simulink model "AERO560_HW6Sim_Thapar"  (R2022b)
settings: Solver=VariableStepAuto  StartTime=0.0  StopTime=10.0  RelTol=1e-3
undefined symbols (not defined in the file): p1, seed
settings Model: Creator=gagandeepthapar  LastModifiedBy=gagandeepthapar

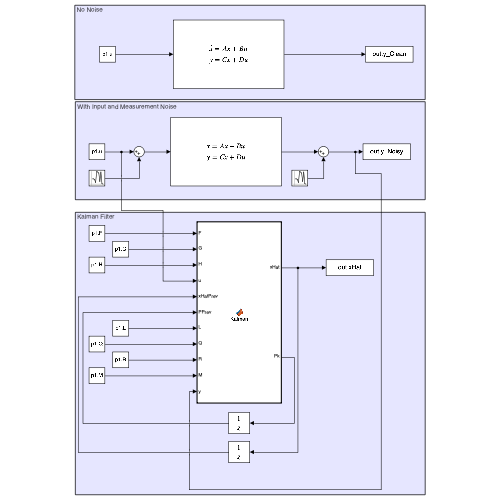
[thumbnail: Simulink's stored preview of the top-level diagram]
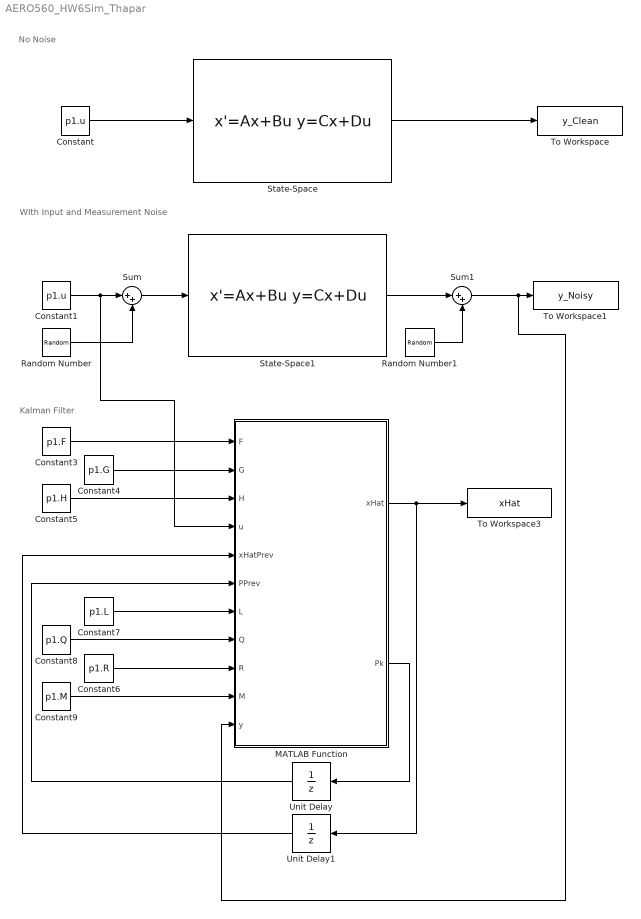
== system AERO560_HW6Sim_Thapar ==
  note: WIth Input and Measurement Noise
  note: No Noise
  note: Kalman Filter
  Constant : Constant  Value=p1.u  VectorParams1D=off
  Constant1 : Constant  Value=p1.u  VectorParams1D=off
  Constant3 : Constant  Value=p1.F  VectorParams1D=off
  Constant4 : Constant  Value=p1.G  VectorParams1D=off
  Constant5 : Constant  Value=p1.H  VectorParams1D=off
  Constant6 : Constant  Value=p1.R  VectorParams1D=off
  Constant7 : Constant  Value=p1.L  VectorParams1D=off
  Constant8 : Constant  Value=p1.Q  VectorParams1D=off
  Constant9 : Constant  Value=p1.M  VectorParams1D=off
  MATLAB Function : MATLAB Function  TreatAsAtomicUnit=on
  Random Number : RandomNumber  Variance=p1.sigma^2  Seed=seed  SampleTime=p1.delT
  Random Number1 : RandomNumber  Variance=p1.sigma^2  Seed=seed+2  SampleTime=p1.delT
  State-Space : StateSpace  A=p1.A  B=p1.B  C=p1.C  D=p1.D  InitialCondition=p1.state0
  State-Space1 : StateSpace  A=p1.A  B=p1.B  C=p1.C  D=p1.D  InitialCondition=p1.state0
  Sum : Sum  Inputs=|++
  Sum1 : Sum  Inputs=|++
  To Workspace : ToWorkspace  VariableName=y_Clean  SampleTime=-1
      settings: Save2DSignal=2-D array (concatenate along first dimension)
  To Workspace1 : ToWorkspace  VariableName=y_Noisy  SampleTime=-1
      settings: Save2DSignal=2-D array (concatenate along first dimension)
  To Workspace3 : ToWorkspace  VariableName=xHat  SampleTime=-1
      settings: Save2DSignal=2-D array (concatenate along first dimension)
  Unit Delay : UnitDelay  SampleTime=-1  HasFrameUpgradeWarning=on
  Unit Delay1 : UnitDelay  InitialCondition=p1.state0  SampleTime=-1  HasFrameUpgradeWarning=on
  wires:
  State-Space/1 -> To Workspace/1
  Constant/1 -> State-Space/1
  Constant1/1 -> MATLAB Function/4(u), Sum/1
  Sum/1 -> State-Space1/1
  Random Number/1 -> Sum/2
  State-Space1/1 -> Sum1/1
  Random Number1/1 -> Sum1/2
  Constant3/1 -> MATLAB Function/1(F)
  Constant4/1 -> MATLAB Function/2(G)
  Constant5/1 -> MATLAB Function/3(H)
  Constant7/1 -> MATLAB Function/7(L)
  Constant8/1 -> MATLAB Function/8(Q)
  Constant6/1 -> MATLAB Function/9(R)
  Constant9/1 -> MATLAB Function/10(M)
  MATLAB Function/2(Pk) -> Unit Delay/1
  MATLAB Function/1(xHat) -> To Workspace3/1, Unit Delay1/1
  Unit Delay1/1 -> MATLAB Function/5(xHatPrev)
  Unit Delay/1 -> MATLAB Function/6(PPrev)
  Sum1/1 -> To Workspace1/1, MATLAB Function/11(y)

== matlab function AERO560_HW6Sim_Thapar/MATLAB Function ==
  data: F input; G input; H input; u input; xHat output; Pk output; xHatPrev input; PPrev input; L input; Q input; R input; M input; y input
function [xHat, Pk] = Kalman(F, G, H, u, xHatPrev, PPrev, L, Q, R, M, y)

% predictor
xHatMinus = F*xHatPrev + G*u;
PkMinus = F*PPrev*F' + L*Q*L';

% corrector
W = H*PkMinus*H' + M*R*M';
K = PkMinus * H' * inv(W);

yHatMinus = H*xHatMinus;

xHat = xHatMinus + K*(y - yHatMinus);
Pk = PkMinus - K*H*PkMinus - PkMinus*H'*K' + K*W*K';

end
